simulink model "EScooter_Functional_Architecture"  (R2025b)
settings: Solver=VariableStepAuto  StartTime=0.0  StopTime=10.0  RelTol=1e-3
settings Model: Creator=louis  LastModifiedBy=louis

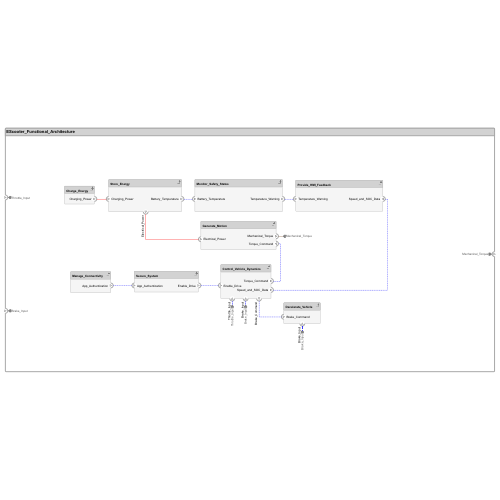
[thumbnail: Simulink's stored preview of the top-level diagram]
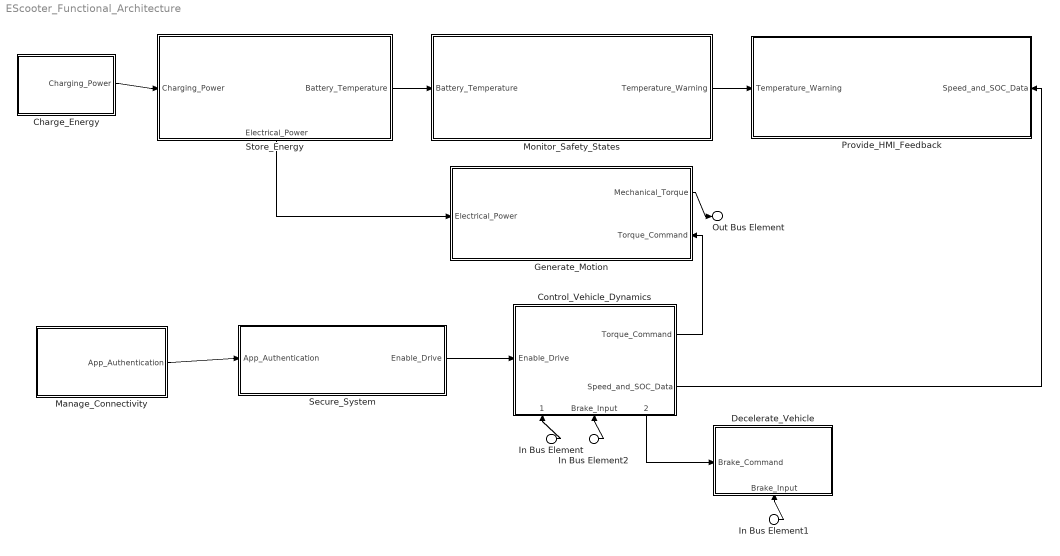
== system EScooter_Functional_Architecture ==
  In Bus Element : Inport  PortName=Throttle_Input
  In Bus Element1 : Inport  Port=2  PortName=Brake_Input
  In Bus Element2 : Inport  Port=2  PortName=Brake_Input
  Charge_Energy : Subsystem
      settings: PortSchema="{\"entries\":[{\"content\":{\"headerSize\":26,\"margin\":15,\"minimumSpacing\":25,\"sides\":[{\"content\":{},\"type\":\"ConnectorPlacement.EquallySpacedRectSide\",\"uuid\":\"e142a197-65ba-49f5-984e-f122eaf5d044\"},{\"content\":{\"connectorIds\":[\"Out1\"],\"side\":\"RIGHT\"},\"type\":\"ConnectorPlacement.EquallySpacedRectSide\",\"uuid\":\"1fdc192c-7e17-4f29-a444-2a532083eda5\"},{\"content\":{\"side\":\"TOP\"},\"type\":\"ConnectorPlacement.EquallySpacedRectSide\",\"uuid\":\"69d74a18-4469-4364-b50f-85fa2c4ecf23\"}]},\"type\":\"ConnectorPlacement.EquallySpacedConnector\",\"uuid\":\"0a196daf-1b77-4056-b99e-f6997ad8671f\"}],\"packageUris\":[\"http://schema.mathworks.com/mf0/Connector/R2020b\"],\"version\":\"1.0\"}"
  Control_Vehicle_Dynamics : Subsystem
      settings: PortSchema="{\"entries\":[{\"content\":{\"headerSize\":26,\"margin\":15,\"minimumSpacing\":25,\"sides\":[{\"content\":{\"connectorIds\":[\"In3\"]},\"type\":\"ConnectorPlacement.EquallySpacedRectSide\",\"uuid\":\"e142a197-65ba-49f5-984e-f122eaf5d044\"},{\"content\":{\"connectorIds\":[\"Out3\",\"Out1\"],\"side\":\"RIGHT\"},\"type\":\"ConnectorPlacement.EquallySpacedRectSide\",\"uuid\":\"1fdc192c-7e17-4f29-a444-2a532083eda5\"},{\"content\":{\"side\":\"TOP\"},\"type\":\"ConnectorPlacement.EquallySpacedRectSide\",\"uuid\":\"69d74a18-4469-4364-b50f-85fa2c4ecf23\"},{\"content\":{\"connectorIds\":[\"In1\",\"In2\",\"Out2\"],\"side\":\"BOTTOM\"},\"type\":\"ConnectorPlacement.EquallySpacedRectSide\",\"uuid\":\"661b6b46-a76e-428b-a8b6-4ba7d3c01746\"}]},\"type\":\"ConnectorPlacement.EquallySpacedConnector\",\"uuid\":\"0a196daf-1b77-4056-b99e-f6997ad8671f\"}],\"packageUris\":[\"http://schema.mathworks.com/mf0/Connector/R2020b\"],\"version\":\"1.0\"}"
  Decelerate_Vehicle : Subsystem
      settings: PortSchema="{\"entries\":[{\"content\":{\"headerSize\":26,\"margin\":15,\"minimumSpacing\":25,\"sides\":[{\"content\":{\"connectorIds\":[\"In2\"]},\"type\":\"ConnectorPlacement.EquallySpacedRectSide\",\"uuid\":\"e142a197-65ba-49f5-984e-f122eaf5d044\"},{\"content\":{\"side\":\"RIGHT\"},\"type\":\"ConnectorPlacement.EquallySpacedRectSide\",\"uuid\":\"1fdc192c-7e17-4f29-a444-2a532083eda5\"},{\"content\":{\"side\":\"TOP\"},\"type\":\"ConnectorPlacement.EquallySpacedRectSide\",\"uuid\":\"69d74a18-4469-4364-b50f-85fa2c4ecf23\"},{\"content\":{\"connectorIds\":[\"In1\"],\"side\":\"BOTTOM\"},\"type\":\"ConnectorPlacement.EquallySpacedRectSide\",\"uuid\":\"0506b342-235d-4893-8dcd-17775360b220\"}]},\"type\":\"ConnectorPlacement.EquallySpacedConnector\",\"uuid\":\"0a196daf-1b77-4056-b99e-f6997ad8671f\"}],\"packageUris\":[\"http://schema.mathworks.com/mf0/Connector/R2020b\"],\"version\":\"1.0\"}"
  Generate_Motion : Subsystem
      settings: PortSchema="{\"entries\":[{\"content\":{\"headerSize\":26,\"margin\":15,\"minimumSpacing\":25,\"sides\":[{\"content\":{\"connectorIds\":[\"In2\"]},\"type\":\"ConnectorPlacement.EquallySpacedRectSide\",\"uuid\":\"e142a197-65ba-49f5-984e-f122eaf5d044\"},{\"content\":{\"connectorIds\":[\"Out1\",\"In1\"],\"side\":\"RIGHT\"},\"type\":\"ConnectorPlacement.EquallySpacedRectSide\",\"uuid\":\"1fdc192c-7e17-4f29-a444-2a532083eda5\"},{\"content\":{\"side\":\"TOP\"},\"type\":\"ConnectorPlacement.EquallySpacedRectSide\",\"uuid\":\"69d74a18-4469-4364-b50f-85fa2c4ecf23\"},{\"content\":{\"side\":\"BOTTOM\"},\"type\":\"ConnectorPlacement.EquallySpacedRectSide\",\"uuid\":\"2c13b6b3-4a8f-4c4b-9699-e14aba2dc0a3\"}]},\"type\":\"ConnectorPlacement.EquallySpacedConnector\",\"uuid\":\"0a196daf-1b77-4056-b99e-f6997ad8671f\"}],\"packageUris\":[\"http://schema.mathworks.com/mf0/Connector/R2020b\"],\"version\":\"1.0\"}"
  Manage_Connectivity : Subsystem
      settings: PortSchema="{\"entries\":[{\"content\":{\"headerSize\":26,\"margin\":15,\"minimumSpacing\":25,\"sides\":[{\"content\":{},\"type\":\"ConnectorPlacement.EquallySpacedRectSide\",\"uuid\":\"e142a197-65ba-49f5-984e-f122eaf5d044\"},{\"content\":{\"connectorIds\":[\"Out1\"],\"side\":\"RIGHT\"},\"type\":\"ConnectorPlacement.EquallySpacedRectSide\",\"uuid\":\"1fdc192c-7e17-4f29-a444-2a532083eda5\"},{\"content\":{\"side\":\"TOP\"},\"type\":\"ConnectorPlacement.EquallySpacedRectSide\",\"uuid\":\"69d74a18-4469-4364-b50f-85fa2c4ecf23\"}]},\"type\":\"ConnectorPlacement.EquallySpacedConnector\",\"uuid\":\"0a196daf-1b77-4056-b99e-f6997ad8671f\"}],\"packageUris\":[\"http://schema.mathworks.com/mf0/Connector/R2020b\"],\"version\":\"1.0\"}"
  Monitor_Safety_States : Subsystem
      settings: PortSchema="{\"entries\":[{\"content\":{\"headerSize\":26,\"margin\":15,\"minimumSpacing\":25,\"sides\":[{\"content\":{\"connectorIds\":[\"In1\"]},\"type\":\"ConnectorPlacement.EquallySpacedRectSide\",\"uuid\":\"e142a197-65ba-49f5-984e-f122eaf5d044\"},{\"content\":{\"connectorIds\":[\"Out1\"],\"side\":\"RIGHT\"},\"type\":\"ConnectorPlacement.EquallySpacedRectSide\",\"uuid\":\"1fdc192c-7e17-4f29-a444-2a532083eda5\"},{\"content\":{\"side\":\"TOP\"},\"type\":\"ConnectorPlacement.EquallySpacedRectSide\",\"uuid\":\"69d74a18-4469-4364-b50f-85fa2c4ecf23\"},{\"content\":{\"side\":\"BOTTOM\"},\"type\":\"ConnectorPlacement.EquallySpacedRectSide\",\"uuid\":\"9bedad61-c0a3-46b7-86fc-b1381f3e3371\"}]},\"type\":\"ConnectorPlacement.EquallySpacedConnector\",\"uuid\":\"0a196daf-1b77-4056-b99e-f6997ad8671f\"}],\"packageUris\":[\"http://schema.mathworks.com/mf0/Connector/R2020b\"],\"version\":\"1.0\"}"
  Provide_HMI_Feedback : Subsystem
      settings: PortSchema="{\"entries\":[{\"content\":{\"headerSize\":26,\"margin\":15,\"minimumSpacing\":25,\"sides\":[{\"content\":{\"connectorIds\":[\"In2\"]},\"type\":\"ConnectorPlacement.EquallySpacedRectSide\",\"uuid\":\"e142a197-65ba-49f5-984e-f122eaf5d044\"},{\"content\":{\"connectorIds\":[\"In1\"],\"side\":\"RIGHT\"},\"type\":\"ConnectorPlacement.EquallySpacedRectSide\",\"uuid\":\"1fdc192c-7e17-4f29-a444-2a532083eda5\"},{\"content\":{\"side\":\"TOP\"},\"type\":\"ConnectorPlacement.EquallySpacedRectSide\",\"uuid\":\"69d74a18-4469-4364-b50f-85fa2c4ecf23\"},{\"content\":{\"side\":\"BOTTOM\"},\"type\":\"ConnectorPlacement.EquallySpacedRectSide\",\"uuid\":\"751cb111-1596-45e6-b236-d28b8d929d55\"}]},\"type\":\"ConnectorPlacement.EquallySpacedConnector\",\"uuid\":\"0a196daf-1b77-4056-b99e-f6997ad8671f\"}],\"packageUris\":[\"http://schema.mathworks.com/mf0/Connector/R2020b\"],\"version\":\"1.0\"}"
  Secure_System : Subsystem
      settings: PortSchema="{\"entries\":[{\"content\":{\"headerSize\":26,\"margin\":15,\"minimumSpacing\":25,\"sides\":[{\"content\":{\"connectorIds\":[\"In1\"]},\"type\":\"ConnectorPlacement.EquallySpacedRectSide\",\"uuid\":\"e142a197-65ba-49f5-984e-f122eaf5d044\"},{\"content\":{\"connectorIds\":[\"Out1\"],\"side\":\"RIGHT\"},\"type\":\"ConnectorPlacement.EquallySpacedRectSide\",\"uuid\":\"1fdc192c-7e17-4f29-a444-2a532083eda5\"},{\"content\":{\"side\":\"TOP\"},\"type\":\"ConnectorPlacement.EquallySpacedRectSide\",\"uuid\":\"69d74a18-4469-4364-b50f-85fa2c4ecf23\"}]},\"type\":\"ConnectorPlacement.EquallySpacedConnector\",\"uuid\":\"0a196daf-1b77-4056-b99e-f6997ad8671f\"}],\"packageUris\":[\"http://schema.mathworks.com/mf0/Connector/R2020b\"],\"version\":\"1.0\"}"
  Store_Energy : Subsystem
      settings: PortSchema="{\"entries\":[{\"content\":{\"headerSize\":26,\"margin\":15,\"minimumSpacing\":25,\"sides\":[{\"content\":{\"connectorIds\":[\"In1\"]},\"type\":\"ConnectorPlacement.EquallySpacedRectSide\",\"uuid\":\"e142a197-65ba-49f5-984e-f122eaf5d044\"},{\"content\":{\"connectorIds\":[\"Out1\"],\"side\":\"RIGHT\"},\"type\":\"ConnectorPlacement.EquallySpacedRectSide\",\"uuid\":\"1fdc192c-7e17-4f29-a444-2a532083eda5\"},{\"content\":{\"side\":\"TOP\"},\"type\":\"ConnectorPlacement.EquallySpacedRectSide\",\"uuid\":\"69d74a18-4469-4364-b50f-85fa2c4ecf23\"},{\"content\":{\"connectorIds\":[\"Out2\"],\"side\":\"BOTTOM\"},\"type\":\"ConnectorPlacement.EquallySpacedRectSide\",\"uuid\":\"55545aa3-ffbe-4d26-961a-543023c7adbb\"}]},\"type\":\"ConnectorPlacement.EquallySpacedConnector\",\"uuid\":\"0a196daf-1b77-4056-b99e-f6997ad8671f\"}],\"packageUris\":[\"http://schema.mathworks.com/mf0/Connector/R2020b\"],\"version\":\"1.0\"}"
  Out Bus Element : Outport  PortName=Mechanical_Torque
  wires:
  Manage_Connectivity/1(App_Authentication) -> Secure_System/1(App_Authentication)
  Monitor_Safety_States/1(Temperature_Warning) -> Provide_HMI_Feedback/2(Temperature_Warning)
  Secure_System/1(Enable_Drive) -> Control_Vehicle_Dynamics/3(Enable_Drive)
  Charge_Energy/1(Charging_Power) -> Store_Energy/1(Charging_Power)
  Store_Energy/1(Battery_Temperature) -> Monitor_Safety_States/1(Battery_Temperature)
  Store_Energy/2(Electrical_Power) -> Generate_Motion/2(Electrical_Power)
  Control_Vehicle_Dynamics/1(Speed_and_SOC_Data) -> Provide_HMI_Feedback/1(Speed_and_SOC_Data)
  Control_Vehicle_Dynamics/2(Brake_Command) -> Decelerate_Vehicle/2(Brake_Command)
  Control_Vehicle_Dynamics/3(Torque_Command) -> Generate_Motion/1(Torque_Command)
  Generate_Motion/1(Mechanical_Torque) -> Out Bus Element/1
  In Bus Element/1 -> Control_Vehicle_Dynamics/1(Throttle_Input)
  In Bus Element1/1 -> Decelerate_Vehicle/1(Brake_Input)
  In Bus Element2/1 -> Control_Vehicle_Dynamics/2(Brake_Input)

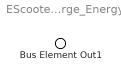
== system EScooter_Functional_Architecture/Charge_Energy ==
  Bus Element Out1 : Outport  PortName=Charging_Power

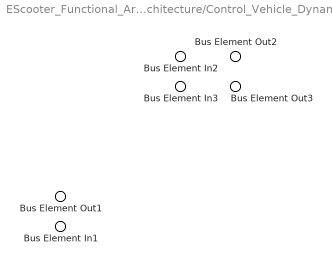
== system EScooter_Functional_Architecture/Control_Vehicle_Dynamics ==
  Bus Element In2 : Inport  PortName=Throttle_Input
  Bus Element In3 : Inport  Port=2  PortName=Brake_Input
  Bus Element In1 : Inport  Port=3  PortName=Enable_Drive
  Bus Element Out3 : Outport  PortName=Speed_and_SOC_Data
  Bus Element Out2 : Outport  Port=2  PortName=Brake_Command
  Bus Element Out1 : Outport  Port=3  PortName=Torque_Command

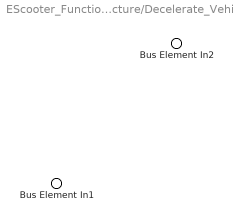
== system EScooter_Functional_Architecture/Decelerate_Vehicle ==
  Bus Element In2 : Inport  PortName=Brake_Input
  Bus Element In1 : Inport  Port=2  PortName=Brake_Command

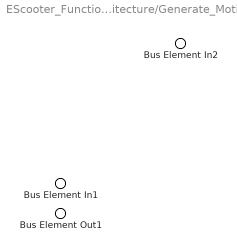
== system EScooter_Functional_Architecture/Generate_Motion ==
  Bus Element In2 : Inport  PortName=Torque_Command
  Bus Element In1 : Inport  Port=2  PortName=Electrical_Power
  Bus Element Out1 : Outport  PortName=Mechanical_Torque

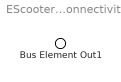
== system EScooter_Functional_Architecture/Manage_Connectivity ==
  Bus Element Out1 : Outport  PortName=App_Authentication

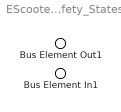
== system EScooter_Functional_Architecture/Monitor_Safety_States ==
  Bus Element In1 : Inport  PortName=Battery_Temperature
  Bus Element Out1 : Outport  PortName=Temperature_Warning

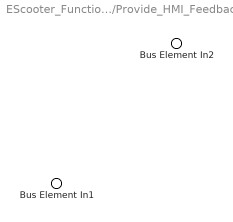
== system EScooter_Functional_Architecture/Provide_HMI_Feedback ==
  Bus Element In2 : Inport  PortName=Speed_and_SOC_Data
  Bus Element In1 : Inport  Port=2  PortName=Temperature_Warning

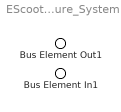
== system EScooter_Functional_Architecture/Secure_System ==
  Bus Element In1 : Inport  PortName=App_Authentication
  Bus Element Out1 : Outport  PortName=Enable_Drive

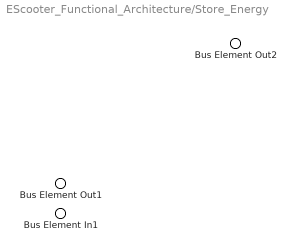
== system EScooter_Functional_Architecture/Store_Energy ==
  Bus Element In1 : Inport  PortName=Charging_Power
  Bus Element Out2 : Outport  PortName=Battery_Temperature
  Bus Element Out1 : Outport  Port=2  PortName=Electrical_Power
